simulink model "task2f"  (R2016a)
settings: Solver=VariableStepAuto  StartTime=0.0  StopTime=100.0  RelTol=1e-3
values from neighbouring files (symbols this model uses):
  A = [[-0.322 0.052 0.028 -1.12 0.002] ... (first row only)    [Ass_2_ailerons.m]
  g = 9.81    [Ass_2_ailerons.m]
  kd = (2*zeta_phi*omega_n-a1)/a2    [Ass_2_ailerons.m]
  ki = 0.85    [Ass_2_ailerons.m]
  kp = 2*sign(a2)    [Ass_2_ailerons.m]
  kp_x = 7.5    [Ass_2_ailerons.m]
  Vg = 580/3.6    (= 161.111111111)    [Ass_2_ailerons.m]
settings Model: Creator=magnusschmidt  LastModifiedBy=magnusschmidt

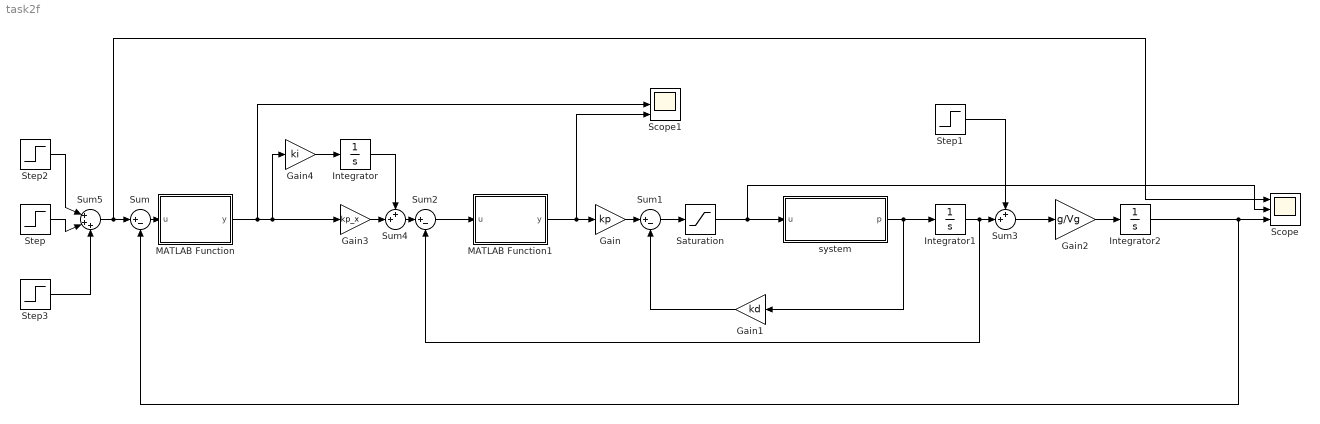
== system task2f ==
  Gain : Gain  Gain=kp
  Gain1 : Gain  Gain=kd
  Gain2 : Gain  Gain=g/Vg
  Gain3 : Gain  Gain=kp_x
  Gain4 : Gain  Gain=ki
  Integrator : Integrator
  Integrator1 : Integrator
  Integrator2 : Integrator
  MATLAB Function : MATLAB Function  TreatAsAtomicUnit=on
  MATLAB Function1 : MATLAB Function  TreatAsAtomicUnit=on
  Saturation : Saturate  UpperLimit=30  LowerLimit=-30
  Scope : Scope  NumInputPorts=3
  Scope1 : Scope  NumInputPorts=3
  Step : Step  Time=35  After=-5  SampleTime=0
  Step1 : Step  Time=0  After=1.5  SampleTime=0
  Step2 : Step  Time=10  After=5  SampleTime=0
  Step3 : Step  Time=65  After=5  SampleTime=0
  Sum : Sum  Inputs=|+-
  Sum1 : Sum  Inputs=|+-
  Sum2 : Sum  Inputs=|+-
  Sum3 : Sum  Inputs=++|
  Sum4 : Sum  Inputs=++|
  Sum5 : Sum  Inputs=|+++
  system : Subsystem
  wires:
  system/1(p) -> Gain1/1, Integrator1/1
  Gain1/1 -> Sum1/2
  Gain/1 -> Sum1/1
  Sum2/1 -> MATLAB Function1/1(u)
  Integrator1/1 -> Sum3/2, Sum2/2
  Sum3/1 -> Gain2/1
  Gain2/1 -> Integrator2/1
  Step1/1 -> Sum3/1
  Sum4/1 -> Sum2/1
  Gain3/1 -> Sum4/2
  Gain4/1 -> Integrator/1
  Integrator/1 -> Sum4/1
  Integrator2/1 -> Scope/3, Sum/2
  Sum5/1 -> Scope/1, Sum/1
  Step2/1 -> Sum5/1
  Step/1 -> Sum5/2
  Step3/1 -> Sum5/3
  Sum1/1 -> Saturation/1
  Saturation/1 -> system/1(u), Scope/2
  MATLAB Function/1(y) -> Scope1/2, Gain3/1, Gain4/1
  MATLAB Function1/1(y) -> Scope1/3, Gain/1
  Sum/1 -> MATLAB Function/1(u)

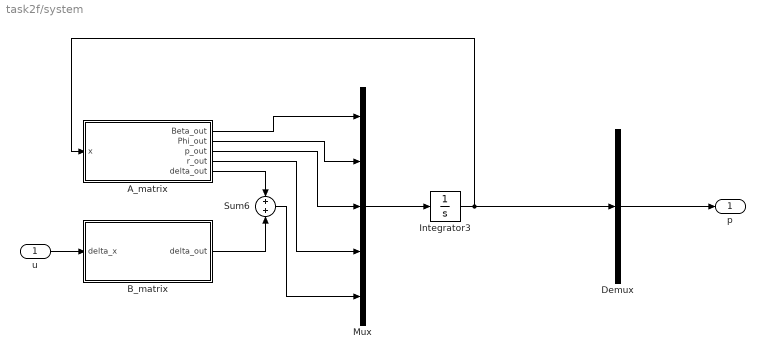
== system task2f/system ==
  u : Inport
  A_matrix : Subsystem
  B_matrix : Subsystem
  Demux : Demux  Outputs=5
  Integrator3 : Integrator
  Mux : Mux  Inputs=5
  Sum6 : Sum
  p : Outport
  wires:
  A_matrix/5(delta_out) -> Sum6/1
  B_matrix/1(delta_out) -> Sum6/2
  A_matrix/1(Beta_out) -> Mux/1
  A_matrix/3(p_out) -> Mux/3
  A_matrix/4(r_out) -> Mux/4
  A_matrix/2(Phi_out) -> Mux/2
  Sum6/1 -> Mux/5
  Mux/1 -> Integrator3/1
  Integrator3/1 -> Demux/1, A_matrix/1(x)
  u/1 -> B_matrix/1(delta_x)
  Demux/3 -> p/1

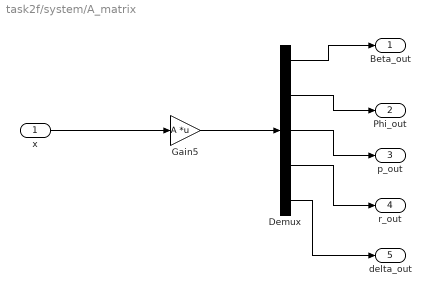
== system task2f/system/A_matrix ==
  x : Inport
  Demux : Demux  Outputs=5
  Gain5 : Gain  Gain=A  Multiplication=Matrix(K*u) (u vector)
  Beta_out : Outport
  Phi_out : Outport  Port=2
  p_out : Outport  Port=3
  r_out : Outport  Port=4
  delta_out : Outport  Port=5
  wires:
  Gain5/1 -> Demux/1
  Demux/1 -> Beta_out/1
  Demux/2 -> Phi_out/1
  Demux/3 -> p_out/1
  Demux/4 -> r_out/1
  Demux/5 -> delta_out/1
  x/1 -> Gain5/1

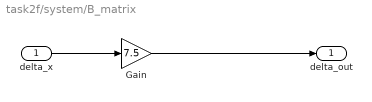
== system task2f/system/B_matrix ==
  delta_x : Inport
  Gain : Gain  Gain=7.5
  delta_out : Outport
  wires:
  delta_x/1 -> Gain/1
  Gain/1 -> delta_out/1

== matlab function task2f/MATLAB Function1 ==
  data: u input; y output
function y = fcn(u)

y = mod(u+180,360)-180;

== matlab function task2f/MATLAB Function ==
  data: u input; y output
function y = fcn(u)

y = mod(u+180,360)-180;
